simulink model "step_PID"  (R2017a)
settings: Solver=ode45  StartTime=0.0  StopTime=50  MaxStep=1e-3  RelTol=1e-3  EnableMultiTasking=on
undefined symbols (not defined in the file or in its folder): p, sigbuilder_block
libraries: simulink x45, cstblocks x3
settings Model: Creator=jmgomes  LastModifiedBy=guir
settings DataIOCC: SaveFormat=Array  SignalLoggingSaveFormat=ModelDataLogs
settings OptimizationCC: ExpressionDepthLimit=2147483647  InitFltsAndDblsToZero=on  LifeSpan=inf
settings DebuggingCC: SaveWithParameterizedLinksMsg=none  UnderspecifiedInitializationDetection=Classic  MergeDetectMultiDrivingBlocksExec=none  SignalResolutionControl=TryResolveAllWithWarning  SolverPrmCheckMsg=warning  MultiTaskDSMMsg=warning  MultiTaskCondExecSysMsg=none  FcnCallInpInsideContextMsg=warning  StateNameClashWarn=warning  SFUnexpectedBacktrackingDiag=warning  SFNoUnconditionalDefaultTransitionDiag=warning  SFExecutionAtInitializationDiag=none
settings HardwareCC: ProdBitPerPointer=32  ProdBitPerSizeT=32  ProdBitPerPtrDiffT=32  ProdLargestAtomicFloat=None  ProdIntDivRoundTo=Undefined  ProdEndianess=Unspecified  ProdWordSize=32  ProdHWDeviceType=32-bit Generic
settings ModelReferenceCC: PropagateSignalLabelsOutOfModel=off
settings GRTTargetCC: TargetFcnLib=ansi_tfl_tmw.mat  TargetLangStandard=C89/C90 (ANSI)  GeneratePreprocessorConditionals=Disable all  CombineOutputUpdateFcns=off  GRTInterface=on
settings ConfigComp: CovMetricSettings=dw  CovHtmlReporting=on  CovSaveCumulativeToWorkspaceVar=on  CovSaveSingleToWorkspaceVar=on  CovExternalEMLEnable=off

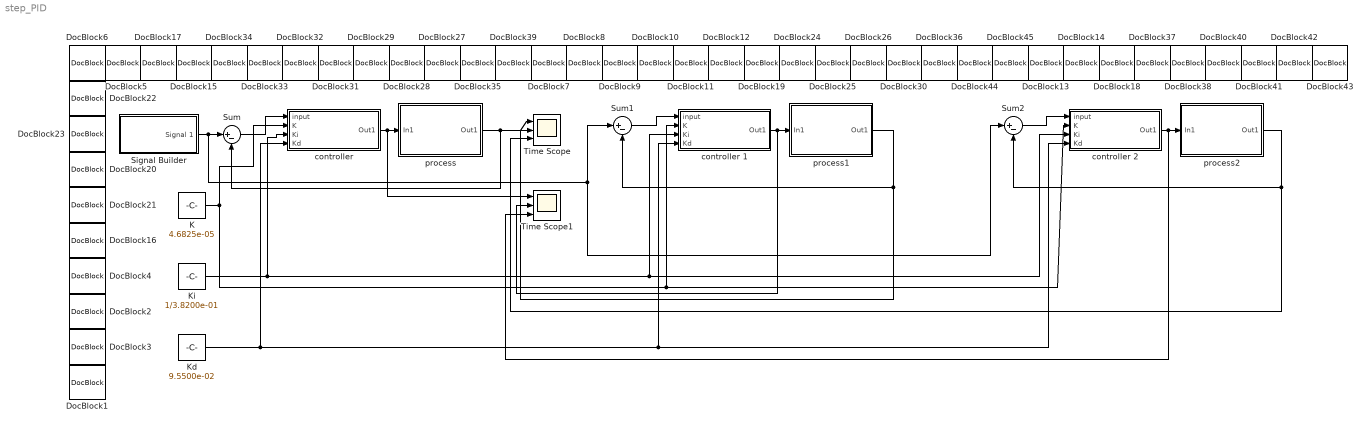
== system step_PID ==
  DocBlock{1..45} (45 alike) : simulink/Model-Wide Utilities/DocBlock  DocumentType=Text
      content=|
      | Type your documentation here
  K : Constant  Value=4.6825e-05
  Kd : Constant  Value=9.5500e-02
  Ki : Constant  Value=1/3.8200e-01
  Signal Builder : Subsystem  Tag=STV Subsys  LoadFcn=sigbuilder_block('load');  StartFcn=sigbuilder_block('start');  StopFcn=sigbuilder_block('stop');  ClipboardFcn=sigbuilder_block('clipboard');  mask(Sigbuilder block){tuvar=[0:10]}
      mask help: Simulink:masks:SigbuilderBlock_MD
      mask init:
      | if ~strcmp(get_param(bdroot(gcbh),'SimulationStatus'),'stopped') tuvar = sigbuilder_block('maskInit'); end
      settings: CopyFcn=sigbuilder_block('copy');  DeleteFcn=sigbuilder_block('delete');  ModelCloseFcn=sigbuilder_block('modelClose');  PreSaveFcn=sigbuilder_block('preSave');  PauseFcn=sigbuilder_block('pause');  ContinueFcn=sigbuilder_block('continue');  NameChangeFcn=sigbuilder_block('namechange');  OpenFcn=sigbuilder_block('open',[0 23.25 1024.5 489.75 ]);  CloseFcn=sigbuilder_block('close');
      mask Display: plot(0, 0, 100, 100,[2, 2, 32, 32, 2], [68, 8, 8, 68, 68],[32, 2], [38, 38], [32, 19, 2],[53, 60, 44], [32, 17, 17, 2],[16, 16, 31, 31]);txt = getActiveGroup(gcbh);text(2, 100, txt,'verticalAlignment', 'top');
  Sum : Sum  Inputs=|+-
  Sum1 : Sum  Inputs=|+-
  Sum2 : Sum  Inputs=|+-
  Time Scope : Scope  NumInputPorts=3
  Time Scope1 : Scope  NumInputPorts=3
  "controller " : Subsystem
  controller 1 : Subsystem
  controller 2 : Subsystem
  process : Subsystem
  process1 : Subsystem
  process2 : Subsystem
  wires:
  Signal Builder/1(Signal 1) -> Sum2/1, Sum1/1, Sum/1
  process/1(Out1) -> Sum/2, Time Scope/1
  "controller "/1(Out1) -> Time Scope1/1, process/1(In1)
  Sum/1 -> "controller "/1(input)
  K/1 -> controller 2/2(K), controller 1/2(K), "controller "/2(K)
  Ki/1 -> controller 2/3(Ki), controller 1/3(Ki), "controller "/3(Ki)
  Kd/1 -> controller 2/4(Kd), controller 1/4(Kd), "controller "/4(Kd)
  controller 1/1(Out1) -> Time Scope1/2, process1/1(In1)
  process2/1(Out1) -> Time Scope/3, Sum2/2
  controller 2/1(Out1) -> Time Scope1/3, process2/1(In1)
  Sum2/1 -> controller 2/1(input)
  Sum1/1 -> controller 1/1(input)
  process1/1(Out1) -> Time Scope/2, Sum1/2

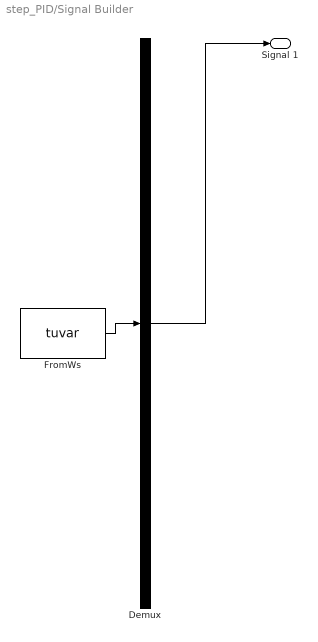
== system step_PID/Signal Builder ==
  Demux : Demux  Tag=STV Demux  Outputs=1
  FromWs : FromWorkspace  Tag=STV FromWs  VariableName=tuvar  SampleTime=0
      SigBuilderData=|
      | common.afterFinalStr = 'Extrapolate'
      | common.sampleTime = 0
      | dataSet.timeRange = [0 50]
      | dataSet.name = 'Group 1'
      | sbobj.Groups.Name = 'Group 1'
      | sbobj.Groups.Signals.Name = 'Signal 1'
      | sbobj.Groups.Signals.XData = [0 25 25 50]
      | sbobj.Groups.Signals.YData = [-300 -300 300 300]
      | sbobj.Groups.TimeRange = [0 50]
  Signal 1 : Outport  Tag=STV Outport
  wires:
  Demux/1 -> Signal 1/1
  FromWs/1 -> Demux/1

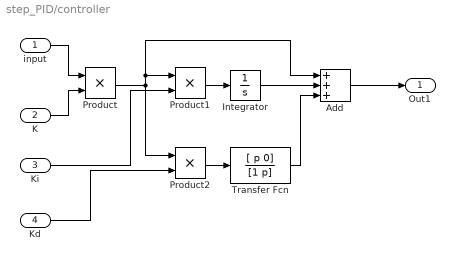
== system step_PID/controller  ==
  input : Inport
  K : Inport  Port=2
  Ki : Inport  Port=3
  Kd : Inport  Port=4
  Add : Sum  Inputs=+++
  Integrator : Integrator
  Product : Product
  Product1 : Product
  Product2 : Product
  Transfer Fcn : TransferFcn  Numerator=[ p 0]  Denominator=[1 p]
  Out1 : Outport
  wires:
  Integrator/1 -> Add/2
  Transfer Fcn/1 -> Add/3
  Product1/1 -> Integrator/1
  Product2/1 -> Transfer Fcn/1
  Product/1 -> Product2/1, Add/1, Product1/1
  input/1 -> Product/1
  Add/1 -> Out1/1
  K/1 -> Product/2
  Ki/1 -> Product1/2
  Kd/1 -> Product2/2

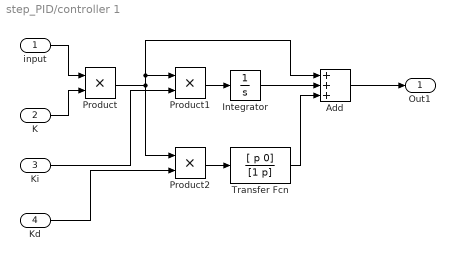
== system step_PID/controller 1 ==
  input : Inport
  K : Inport  Port=2
  Ki : Inport  Port=3
  Kd : Inport  Port=4
  Add : Sum  Inputs=+++
  Integrator : Integrator
  Product : Product
  Product1 : Product
  Product2 : Product
  Transfer Fcn : TransferFcn  Numerator=[ p 0]  Denominator=[1 p]
  Out1 : Outport
  wires:
  Integrator/1 -> Add/2
  Transfer Fcn/1 -> Add/3
  Product1/1 -> Integrator/1
  Product2/1 -> Transfer Fcn/1
  Product/1 -> Product2/1, Add/1, Product1/1
  input/1 -> Product/1
  Add/1 -> Out1/1
  K/1 -> Product/2
  Ki/1 -> Product1/2
  Kd/1 -> Product2/2

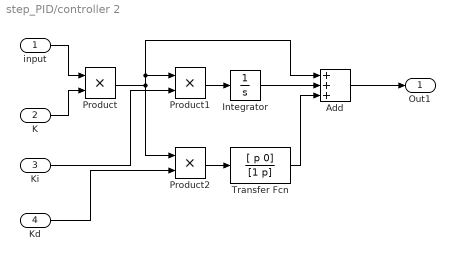
== system step_PID/controller 2 ==
  input : Inport
  K : Inport  Port=2
  Ki : Inport  Port=3
  Kd : Inport  Port=4
  Add : Sum  Inputs=+++
  Integrator : Integrator
  Product : Product
  Product1 : Product
  Product2 : Product
  Transfer Fcn : TransferFcn  Numerator=[ p 0]  Denominator=[1 p]
  Out1 : Outport
  wires:
  Integrator/1 -> Add/2
  Transfer Fcn/1 -> Add/3
  Product1/1 -> Integrator/1
  Product2/1 -> Transfer Fcn/1
  Product/1 -> Product2/1, Add/1, Product1/1
  input/1 -> Product/1
  Add/1 -> Out1/1
  K/1 -> Product/2
  Ki/1 -> Product1/2
  Kd/1 -> Product2/2

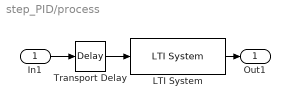
== system step_PID/process ==
  In1 : Inport
  LTI System : cstblocks/LTI System  sys=tfl  IC=[]
  Transport Delay : TransportDelay  DelayTime=0.34
  Out1 : Outport
  wires:
  In1/1 -> Transport Delay/1
  Transport Delay/1 -> LTI System/1
  LTI System/1 -> Out1/1

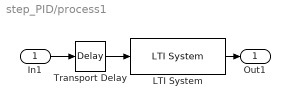
== system step_PID/process1 ==
  In1 : Inport
  LTI System : cstblocks/LTI System  sys=tfb  IC=[]
  Transport Delay : TransportDelay  DelayTime=0.34
  Out1 : Outport
  wires:
  In1/1 -> Transport Delay/1
  Transport Delay/1 -> LTI System/1
  LTI System/1 -> Out1/1

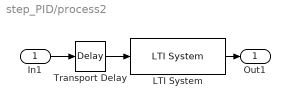
== system step_PID/process2 ==
  In1 : Inport
  LTI System : cstblocks/LTI System  sys=tfr  IC=[]
  Transport Delay : TransportDelay  DelayTime=0.34
  Out1 : Outport
  wires:
  In1/1 -> Transport Delay/1
  Transport Delay/1 -> LTI System/1
  LTI System/1 -> Out1/1
